simulink subsystem "RackAndPinion"  (R2023a)
settings: Solver=VariableStepAuto  StartTime=0.0  StopTime=10.0  RelTol=1e-3
model mask{i_rail=0, M=0, m_pendulum=0, k_visco=0}
  mask prompts: i_rail "Gear ratio of RackAndPinion, [rad/m^3]"; M "Weight of body"; m_pendulum "Weight of inverted pendulum"; k_visco "Coef of viscous friction"
settings Model: Creator=ПК  LastModifiedBy=ПК

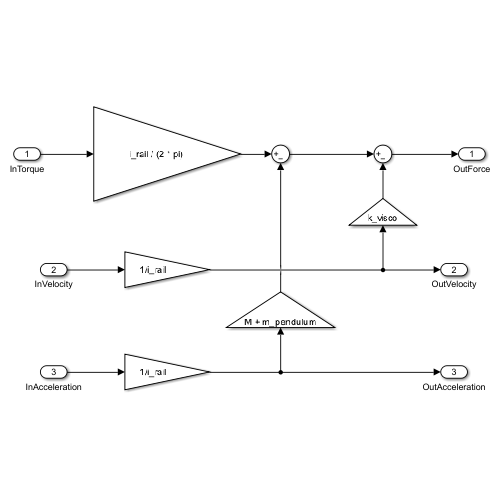
[thumbnail: Simulink's stored preview of the top-level diagram]
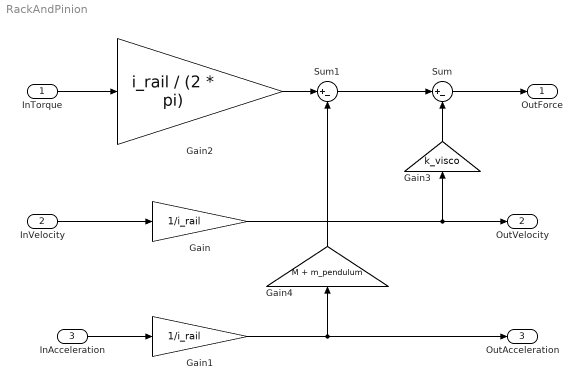
== system RackAndPinion ==
  InTorque : Inport
  InVelocity : Inport  Port=2
  InAcceleration : Inport  Port=3
  Gain : Gain  Gain=1/i_rail
  Gain1 : Gain  Gain=1/i_rail
  Gain2 : Gain  Gain=i_rail / (2 * pi)
  Gain3 : Gain  Gain=k_visco
  Gain4 : Gain  Gain=M + m_pendulum
  Sum : Sum  Inputs=|+-
  Sum1 : Sum  Inputs=|+-
  OutForce : Outport
  OutVelocity : Outport  Port=2
  OutAcceleration : Outport  Port=3
  wires:
  InVelocity/1 -> Gain/1
  Gain/1 -> OutVelocity/1, Gain3/1
  InAcceleration/1 -> Gain1/1
  Gain1/1 -> OutAcceleration/1, Gain4/1
  Gain3/1 -> Sum/2
  Gain2/1 -> Sum1/1
  Sum1/1 -> Sum/1
  Gain4/1 -> Sum1/2
  Sum/1 -> OutForce/1
  InTorque/1 -> Gain2/1
